simulink model "ES105A_StHlthSigNormn"  (R2013b)
settings: Solver=FixedStepDiscrete  SolverMode=SingleTasking  StartTime=0.0  StopTime=1  FixedStep=0.002  RelTol=1e-3
undefined symbols (not defined in the file): ARCHGLBPRM_FLOATZEROTHD_ULS_F32, CurrMeasCorrlnMaxErrCurr, CURRMOTSUMDIVBYZEROPROTNVAL_AMPR_F32, DIGTQDIVBYZEROPROTNVAL_HWNWTMTR_F32, DutyCycThermProtnDutyCycFildThd, EcuTMeasRngDiagcMax, EcuTMeasRngDiagcMin, EotLrngAuthyStrtLrn, FRICESTIMNDIVBYZEROPROTNVAL_HWNWTMTR_F32, HLTH0PERC_CNT_U08, HLTH100PERC_CNT_F32, HLTH100PERC_CNT_U08, HLTH50PERC_CNT_U08, HwTqCorrlnChATraSumSetFltThd, HwTqCorrlnChBTraSumSetFltThd, HWTQIDPTSIG_CNT_U08, MOTAG2MEAS_VALMAXERR_VOLTSQD_F32, MOTAG2MEAS_VALMINERR_VOLTSQD_F32, MOTAGCORRLN_MOTAGCORRLNERRTHD_MOTREVELEC_U0P16, MotDrvDiagcErrThd, MOTPOS2DIVBYZEROPROTNVAL2_VOLTSQD_F32, MOTPOS2DIVBYZEROPROTNVAL_VOLTSQD_F32, MOTPOSNERRDIVBYZEROPROTNVAL_MOTREV_U16, MOTPOSNERRZEROTHD_MOTREV_U0P16, NtcNr1, NtcSts1, PHAVLTGDIVBYZEROPROTNVAL_NANOSEC_F32, SigQlfr1, STHLTHSCAGFAC_CNT_F32, StHlthSigNormnAbsltMotPosDifStHlthDiagThd, StHlthSigNormnCurrMotSumStHlthDiagThd, StHlthSigNormnDigTqStHlthDiagThd, StHlthSigNormnDutyCycFltLimThd, StHlthSigNormnHiCtrlrT, StHlthSigNormnIdptSigStHlthSca, StHlthSigNormnLoCtrlrT, StHlthSigNormnMaxFricThd, StHlthSigNormnMinRackTrvlLim, StHlthSigNormnMotPosStHlthDiagThd, StHlthSigNormnMotVelCal, StHlthSigNormnPhaInfoStHlthDiagThd, StHlthSigNormnStHlthCorrlnErr, StHlthSigNormnStHlthCurrMotSum, StHlthSigNormnStHlthPhaInfo, StHlthSigNormnValMaxStHlthErr, StHlthSigNormnValMinStHlthErr, StHlthSigNormnWhlImbRejctnThd, SysGlbPrmMotPoleCnt, TSTHLTH0PERC_CNT_U08, u2, u3, u4, VLTGSTHLTH0PERC_CNT_U08
libraries: NxtrLim x39, simulink x33, NxtrAbslt x4
(part 7 of 10)

== system ES105A_StHlthSigNormn/StHlthSigNormn/UpdRawSig/Phase Voltage Verification/PhaBStHlth Calc/If Action Subsystem5 ==
  Action Port : ActionPort  ActionType=else
  Constant : Constant  Value=HLTH100PERC_CNT_U08
  CopyRight2 : Subsystem  Description=|  mask(Copyright Information){none=on}
      | Copyright info block.                                               
      |                                                                     
      | Place copyright information at the top of every subsystem in design.
      mask prompts: none "No parameters"
      mask help: Place copyright information at the top of every subsystem in design.
      mask Display:
      | NxtrConf = 'Nexteer Confidential';
      | 
      | sys = bdroot; %handle for the current model ("system")
      | first = get_param(sys,'Created');
      | first = first(end-3:end);  %year is last four digits
      | 
      | last = get_param(sys,'LastModifiedDate');
      | if isempty(last)
      |     last = datestr(now,'yyyy');
      | else
      |     last = last(end-3:end);
      | end
      | 
      | if strcmp(first,last)
      |     fprintf('%s -- Copyright %s Nexteer',NxtrConf,first)
      | else
      |     fprintf('%s -- %s%s- %s Nexteer',NxtrConf,char(169),first,last)
      | end
  PhaseAStHlth : Outport
  wires:
  Constant/1 -> PhaseAStHlth/1

== system ES105A_StHlthSigNormn/StHlthSigNormn/UpdRawSig/Phase Voltage Verification/PhaCStHlth Calc/CopyRight2 ==

== system ES105A_StHlthSigNormn/StHlthSigNormn/UpdRawSig/Phase Voltage Verification/PhaCStHlth Calc/If Action Subsystem8 ==
  MotDrvErrC : Inport
  Action Port : ActionPort  ActionType=then
  Constant : Constant  Value=MotDrvDiagcErrThd
  CopyRight2 : Subsystem  Description=|  mask(Copyright Information){none=on}
      | Copyright info block.                                               
      |                                                                     
      | Place copyright information at the top of every subsystem in design.
      mask prompts: none "No parameters"
      mask help: Place copyright information at the top of every subsystem in design.
      mask Display:
      | NxtrConf = 'Nexteer Confidential';
      | 
      | sys = bdroot; %handle for the current model ("system")
      | first = get_param(sys,'Created');
      | first = first(end-3:end);  %year is last four digits
      | 
      | last = get_param(sys,'LastModifiedDate');
      | if isempty(last)
      |     last = datestr(now,'yyyy');
      | else
      |     last = last(end-3:end);
      | end
      | 
      | if strcmp(first,last)
      |     fprintf('%s -- Copyright %s Nexteer',NxtrConf,first)
      | else
      |     fprintf('%s -- %s%s- %s Nexteer',NxtrConf,char(169),first,last)
      | end
  If : If  IfExpression=u1
  If Action Subsystem : Subsystem  TreatAsAtomicUnit=on
  If Action Subsystem1 : Subsystem  TreatAsAtomicUnit=on
  Merge : Merge
  Relational Operator : RelationalOperator  OutDataTypeStr=boolean
  PhaseCStHlth : Outport
  wires:
  MotDrvErrC/1 -> [MotDrvErrC], Relational Operator/1
  Constant/1 -> Relational Operator/2
  Relational Operator/1 -> If/1
  If/1 -> If Action Subsystem/Action
  If/2 -> If Action Subsystem1/Action
  [MotDrvErrC] -> If Action Subsystem1/1(MotDrvErrC)
  If Action Subsystem/1(PhaseCStHlth) -> Merge/1
  If Action Subsystem1/1(PhaseCStHlth) -> Merge/2
  Merge/1 -> PhaseCStHlth/1

== system ES105A_StHlthSigNormn/StHlthSigNormn/UpdRawSig/Phase Voltage Verification/PhaCStHlth Calc/If Action Subsystem9 ==
  Action Port : ActionPort  ActionType=else
  Constant : Constant  Value=HLTH100PERC_CNT_U08
  CopyRight2 : Subsystem  Description=|  mask(Copyright Information){none=on}
      | Copyright info block.                                               
      |                                                                     
      | Place copyright information at the top of every subsystem in design.
      mask prompts: none "No parameters"
      mask help: Place copyright information at the top of every subsystem in design.
      mask Display:
      | NxtrConf = 'Nexteer Confidential';
      | 
      | sys = bdroot; %handle for the current model ("system")
      | first = get_param(sys,'Created');
      | first = first(end-3:end);  %year is last four digits
      | 
      | last = get_param(sys,'LastModifiedDate');
      | if isempty(last)
      |     last = datestr(now,'yyyy');
      | else
      |     last = last(end-3:end);
      | end
      | 
      | if strcmp(first,last)
      |     fprintf('%s -- Copyright %s Nexteer',NxtrConf,first)
      | else
      |     fprintf('%s -- %s%s- %s Nexteer',NxtrConf,char(169),first,last)
      | end
  PhaseCStHlth : Outport
  wires:
  Constant/1 -> PhaseCStHlth/1

== system ES105A_StHlthSigNormn/StHlthSigNormn/UpdRawSig/Phase Voltage Verification/PhaDStHlth Calc/CopyRight2 ==

== system ES105A_StHlthSigNormn/StHlthSigNormn/UpdRawSig/Phase Voltage Verification/PhaDStHlth Calc/If Action Subsystem12 ==
  MotDrvErrD : Inport
  Action Port : ActionPort  ActionType=then
  Constant : Constant  Value=MotDrvDiagcErrThd
  CopyRight2 : Subsystem  Description=|  mask(Copyright Information){none=on}
      | Copyright info block.                                               
      |                                                                     
      | Place copyright information at the top of every subsystem in design.
      mask prompts: none "No parameters"
      mask help: Place copyright information at the top of every subsystem in design.
      mask Display:
      | NxtrConf = 'Nexteer Confidential';
      | 
      | sys = bdroot; %handle for the current model ("system")
      | first = get_param(sys,'Created');
      | first = first(end-3:end);  %year is last four digits
      | 
      | last = get_param(sys,'LastModifiedDate');
      | if isempty(last)
      |     last = datestr(now,'yyyy');
      | else
      |     last = last(end-3:end);
      | end
      | 
      | if strcmp(first,last)
      |     fprintf('%s -- Copyright %s Nexteer',NxtrConf,first)
      | else
      |     fprintf('%s -- %s%s- %s Nexteer',NxtrConf,char(169),first,last)
      | end
  If : If  IfExpression=u1
  If Action Subsystem : Subsystem  TreatAsAtomicUnit=on
  If Action Subsystem1 : Subsystem  TreatAsAtomicUnit=on
  Merge : Merge
  Relational Operator : RelationalOperator  OutDataTypeStr=boolean
  PhaseDStHlth : Outport
  wires:
  MotDrvErrD/1 -> [MotDrvErrD], Relational Operator/1
  Constant/1 -> Relational Operator/2
  Relational Operator/1 -> If/1
  If/1 -> If Action Subsystem/Action
  If/2 -> If Action Subsystem1/Action
  [MotDrvErrD] -> If Action Subsystem1/1(MotDrvErrD)
  If Action Subsystem/1(PhaseDStHlth) -> Merge/1
  If Action Subsystem1/1(PhaseDStHlth) -> Merge/2
  Merge/1 -> PhaseDStHlth/1

== system ES105A_StHlthSigNormn/StHlthSigNormn/UpdRawSig/Phase Voltage Verification/PhaDStHlth Calc/If Action Subsystem13 ==
  Action Port : ActionPort  ActionType=else
  Constant : Constant  Value=HLTH100PERC_CNT_U08
  CopyRight2 : Subsystem  Description=|  mask(Copyright Information){none=on}
      | Copyright info block.                                               
      |                                                                     
      | Place copyright information at the top of every subsystem in design.
      mask prompts: none "No parameters"
      mask help: Place copyright information at the top of every subsystem in design.
      mask Display:
      | NxtrConf = 'Nexteer Confidential';
      | 
      | sys = bdroot; %handle for the current model ("system")
      | first = get_param(sys,'Created');
      | first = first(end-3:end);  %year is last four digits
      | 
      | last = get_param(sys,'LastModifiedDate');
      | if isempty(last)
      |     last = datestr(now,'yyyy');
      | else
      |     last = last(end-3:end);
      | end
      | 
      | if strcmp(first,last)
      |     fprintf('%s -- Copyright %s Nexteer',NxtrConf,first)
      | else
      |     fprintf('%s -- %s%s- %s Nexteer',NxtrConf,char(169),first,last)
      | end
  PhaseDStHlth : Outport
  wires:
  Constant/1 -> PhaseDStHlth/1

== system ES105A_StHlthSigNormn/StHlthSigNormn/UpdRawSig/Phase Voltage Verification/PhaEStHlth Calc/CopyRight2 ==

== system ES105A_StHlthSigNormn/StHlthSigNormn/UpdRawSig/Phase Voltage Verification/PhaEStHlth Calc/If Action Subsystem16 ==
  MotDrvErrE : Inport
  Action Port : ActionPort  ActionType=then
  Constant : Constant  Value=MotDrvDiagcErrThd
  CopyRight2 : Subsystem  Description=|  mask(Copyright Information){none=on}
      | Copyright info block.                                               
      |                                                                     
      | Place copyright information at the top of every subsystem in design.
      mask prompts: none "No parameters"
      mask help: Place copyright information at the top of every subsystem in design.
      mask Display:
      | NxtrConf = 'Nexteer Confidential';
      | 
      | sys = bdroot; %handle for the current model ("system")
      | first = get_param(sys,'Created');
      | first = first(end-3:end);  %year is last four digits
      | 
      | last = get_param(sys,'LastModifiedDate');
      | if isempty(last)
      |     last = datestr(now,'yyyy');
      | else
      |     last = last(end-3:end);
      | end
      | 
      | if strcmp(first,last)
      |     fprintf('%s -- Copyright %s Nexteer',NxtrConf,first)
      | else
      |     fprintf('%s -- %s%s- %s Nexteer',NxtrConf,char(169),first,last)
      | end
  If : If  IfExpression=u1
  If Action Subsystem : Subsystem  TreatAsAtomicUnit=on
  If Action Subsystem1 : Subsystem  TreatAsAtomicUnit=on
  Merge : Merge
  Relational Operator : RelationalOperator  OutDataTypeStr=boolean
  PhaseEStHlth : Outport
  wires:
  MotDrvErrE/1 -> [MotDrvErrE], Relational Operator/1
  Constant/1 -> Relational Operator/2
  Relational Operator/1 -> If/1
  If/1 -> If Action Subsystem/Action
  If/2 -> If Action Subsystem1/Action
  [MotDrvErrE] -> If Action Subsystem1/1(MotDrvErrE)
  If Action Subsystem/1(PhaseEStHlth) -> Merge/1
  If Action Subsystem1/1(PhaseEStHlth) -> Merge/2
  Merge/1 -> PhaseEStHlth/1

== system ES105A_StHlthSigNormn/StHlthSigNormn/UpdRawSig/Phase Voltage Verification/PhaEStHlth Calc/If Action Subsystem17 ==
  Action Port : ActionPort  ActionType=else
  Constant : Constant  Value=HLTH100PERC_CNT_U08
  CopyRight2 : Subsystem  Description=|  mask(Copyright Information){none=on}
      | Copyright info block.                                               
      |                                                                     
      | Place copyright information at the top of every subsystem in design.
      mask prompts: none "No parameters"
      mask help: Place copyright information at the top of every subsystem in design.
      mask Display:
      | NxtrConf = 'Nexteer Confidential';
      | 
      | sys = bdroot; %handle for the current model ("system")
      | first = get_param(sys,'Created');
      | first = first(end-3:end);  %year is last four digits
      | 
      | last = get_param(sys,'LastModifiedDate');
      | if isempty(last)
      |     last = datestr(now,'yyyy');
      | else
      |     last = last(end-3:end);
      | end
      | 
      | if strcmp(first,last)
      |     fprintf('%s -- Copyright %s Nexteer',NxtrConf,first)
      | else
      |     fprintf('%s -- %s%s- %s Nexteer',NxtrConf,char(169),first,last)
      | end
  PhaseEStHlth : Outport
  wires:
  Constant/1 -> PhaseEStHlth/1

== system ES105A_StHlthSigNormn/StHlthSigNormn/UpdRawSig/Phase Voltage Verification/PhaFStHlth Calc/CopyRight2 ==

== system ES105A_StHlthSigNormn/StHlthSigNormn/UpdRawSig/Phase Voltage Verification/PhaFStHlth Calc/If Action Subsystem20 ==
  MotDrvErrF : Inport
  Action Port : ActionPort  ActionType=then
  Constant : Constant  Value=MotDrvDiagcErrThd
  CopyRight2 : Subsystem  Description=|  mask(Copyright Information){none=on}
      | Copyright info block.                                               
      |                                                                     
      | Place copyright information at the top of every subsystem in design.
      mask prompts: none "No parameters"
      mask help: Place copyright information at the top of every subsystem in design.
      mask Display:
      | NxtrConf = 'Nexteer Confidential';
      | 
      | sys = bdroot; %handle for the current model ("system")
      | first = get_param(sys,'Created');
      | first = first(end-3:end);  %year is last four digits
      | 
      | last = get_param(sys,'LastModifiedDate');
      | if isempty(last)
      |     last = datestr(now,'yyyy');
      | else
      |     last = last(end-3:end);
      | end
      | 
      | if strcmp(first,last)
      |     fprintf('%s -- Copyright %s Nexteer',NxtrConf,first)
      | else
      |     fprintf('%s -- %s%s- %s Nexteer',NxtrConf,char(169),first,last)
      | end
  If : If  IfExpression=u1
  If Action Subsystem : Subsystem  TreatAsAtomicUnit=on
  If Action Subsystem1 : Subsystem  TreatAsAtomicUnit=on
  Merge : Merge
  Relational Operator : RelationalOperator  OutDataTypeStr=boolean
  PhaseFStHlth : Outport
  wires:
  MotDrvErrF/1 -> [MotDrvErrF], Relational Operator/1
  Constant/1 -> Relational Operator/2
  Relational Operator/1 -> If/1
  If/1 -> If Action Subsystem/Action
  If/2 -> If Action Subsystem1/Action
  [MotDrvErrF] -> If Action Subsystem1/1(MotDrvErrF)
  If Action Subsystem/1(PhaseFStHlth) -> Merge/1
  If Action Subsystem1/1(PhaseFStHlth) -> Merge/2
  Merge/1 -> PhaseFStHlth/1

== system ES105A_StHlthSigNormn/StHlthSigNormn/UpdRawSig/Phase Voltage Verification/PhaFStHlth Calc/If Action Subsystem21 ==
  Action Port : ActionPort  ActionType=else
  Constant : Constant  Value=HLTH100PERC_CNT_U08
  CopyRight2 : Subsystem  Description=|  mask(Copyright Information){none=on}
      | Copyright info block.                                               
      |                                                                     
      | Place copyright information at the top of every subsystem in design.
      mask prompts: none "No parameters"
      mask help: Place copyright information at the top of every subsystem in design.
      mask Display:
      | NxtrConf = 'Nexteer Confidential';
      | 
      | sys = bdroot; %handle for the current model ("system")
      | first = get_param(sys,'Created');
      | first = first(end-3:end);  %year is last four digits
      | 
      | last = get_param(sys,'LastModifiedDate');
      | if isempty(last)
      |     last = datestr(now,'yyyy');
      | else
      |     last = last(end-3:end);
      | end
      | 
      | if strcmp(first,last)
      |     fprintf('%s -- Copyright %s Nexteer',NxtrConf,first)
      | else
      |     fprintf('%s -- %s%s- %s Nexteer',NxtrConf,char(169),first,last)
      | end
  PhaseFStHlth : Outport
  wires:
  Constant/1 -> PhaseFStHlth/1

== system ES105A_StHlthSigNormn/StHlthSigNormn/UpdRawSig/Phase Voltage Verification/PhaStHlth/SetNtcSts ==
  note: Note:
      |
      | - "ISO Fault Debounce Design" Simulink block intent to use here for Simulation purpose only. Do not Code this block
  NtcNr : Inport
  NtcStInfo : Inport  Port=2
  NtcSts : Inport  Port=3
  DebStep : Inport  Port=4
  CopyRight2 : Subsystem  Description=|  mask(Copyright Information){none=on}
      | Copyright info block.                                               
      |                                                                     
      | Place copyright information at the top of every subsystem in design.
      mask prompts: none "No parameters"
      mask help: Place copyright information at the top of every subsystem in design.
      mask Display:
      | NxtrConf = 'Nexteer Confidential';
      | 
      | sys = bdroot; %handle for the current model ("system")
      | first = get_param(sys,'Created');
      | first = first(end-3:end);  %year is last four digits
      | 
      | last = get_param(sys,'LastModifiedDate');
      | if isempty(last)
      |     last = datestr(now,'yyyy');
      | else
      |     last = last(end-3:end);
      | end
      | 
      | if strcmp(first,last)
      |     fprintf('%s -- Copyright %s Nexteer',NxtrConf,first)
      | else
      |     fprintf('%s -- %s%s- %s Nexteer',NxtrConf,char(169),first,last)
      | end
  Data Store Write : DataStoreWrite  DataStoreName=NtcQlfr0X1D4
  Ground : Ground
  ISO Fault Debounce Design : Stateflow chart  TreatAsAtomicUnit=on
      settings: AttributesFormatString=|
      | Simulation Purpose Only.
      | Do Not Code this block
      | Diagnostic Manager Owns this requirement
  Terminator : Terminator
  Terminator1 : Terminator
  wires:
  NtcStInfo/1 -> Terminator1/1
  NtcNr/1 -> Terminator/1
  NtcSts/1 -> ISO Fault Debounce Design/1(NtcSts)
  DebStep/1 -> ISO Fault Debounce Design/2(DebStep)
  ISO Fault Debounce Design/1(Qualifier) -> Data Store Write/1
  Ground/1 -> ISO Fault Debounce Design/3(SvcClr)

== system ES105A_StHlthSigNormn/StHlthSigNormn/UpdRawSig/Wheel Imbalance Rejection/If Action Subsystem/CopyRight2 ==

== system ES105A_StHlthSigNormn/StHlthSigNormn/UpdRawSig/Wheel Imbalance Rejection/If Action Subsystem2/CopyRight2 ==

== system ES105A_StHlthSigNormn/StHlthSigNormn/UpdRawSig/ EOT Impact Counter/If Action Subsystem/If Action Subsystem/CopyRight2 ==

== system ES105A_StHlthSigNormn/StHlthSigNormn/UpdRawSig/ EOT Impact Counter/If Action Subsystem/If Action Subsystem/If Action Subsystem ==
  "MotVelCrf " : Inport
  Action Port : ActionPort  ActionType=then
  Constant : Constant  Value=StHlthSigNormnMotVelCal
  CopyRight2 : Subsystem  Description=|  mask(Copyright Information){none=on}
      | Copyright info block.                                               
      |                                                                     
      | Place copyright information at the top of every subsystem in design.
      mask prompts: none "No parameters"
      mask help: Place copyright information at the top of every subsystem in design.
      mask Display:
      | NxtrConf = 'Nexteer Confidential';
      | 
      | sys = bdroot; %handle for the current model ("system")
      | first = get_param(sys,'Created');
      | first = first(end-3:end);  %year is last four digits
      | 
      | last = get_param(sys,'LastModifiedDate');
      | if isempty(last)
      |     last = datestr(now,'yyyy');
      | else
      |     last = last(end-3:end);
      | end
      | 
      | if strcmp(first,last)
      |     fprintf('%s -- Copyright %s Nexteer',NxtrConf,first)
      | else
      |     fprintf('%s -- %s%s- %s Nexteer',NxtrConf,char(169),first,last)
      | end
  Do nothing : Subsystem  TreatAsAtomicUnit=on
  If : If  IfExpression=u1
  If Action Subsystem : Subsystem  TreatAsAtomicUnit=on
  Relational Operator1 : RelationalOperator  Operator=>  OutDataTypeStr=boolean
  wires:
  "MotVelCrf "/1 -> Relational Operator1/1
  Constant/1 -> Relational Operator1/2
  Relational Operator1/1 -> If/1
  If/1 -> If Action Subsystem/Action
  If/2 -> Do nothing/Action

== system ES105A_StHlthSigNormn/StHlthSigNormn/UpdRawSig/ EOT Impact Counter/If Action Subsystem/If Action Subsystem/If Action Subsystem1 ==
  Action Port : ActionPort  ActionType=else
  Constant : Constant  Value=0  OutDataTypeStr=boolean
      settings: AttributesFormatString=%<OutDataTypeStr>
  CopyRight2 : Subsystem  Description=|  mask(Copyright Information){none=on}
      | Copyright info block.                                               
      |                                                                     
      | Place copyright information at the top of every subsystem in design.
      mask prompts: none "No parameters"
      mask help: Place copyright information at the top of every subsystem in design.
      mask Display:
      | NxtrConf = 'Nexteer Confidential';
      | 
      | sys = bdroot; %handle for the current model ("system")
      | first = get_param(sys,'Created');
      | first = first(end-3:end);  %year is last four digits
      | 
      | last = get_param(sys,'LastModifiedDate');
      | if isempty(last)
      |     last = datestr(now,'yyyy');
      | else
      |     last = last(end-3:end);
      | end
      | 
      | if strcmp(first,last)
      |     fprintf('%s -- Copyright %s Nexteer',NxtrConf,first)
      | else
      |     fprintf('%s -- %s%s- %s Nexteer',NxtrConf,char(169),first,last)
      | end
  Data Store Write : DataStoreWrite  DataStoreName=EntrEot
  wires:
  Constant/1 -> Data Store Write/1

== system ES105A_StHlthSigNormn/StHlthSigNormn/UpdRawSig/ EOT Impact Counter/If Action Subsystem/If Action Subsystem1/CopyRight2 ==

== system ES105A_StHlthSigNormn/StHlthSigNormn/UpdRawSig/ EOT Impact Counter/If Action Subsystem/If Action Subsystem1/If Action Subsystem ==
  "MotVelCrf " : Inport
  Action Port : ActionPort  ActionType=then
  Constant : Constant  Value=StHlthSigNormnMotVelCal
  CopyRight2 : Subsystem  Description=|  mask(Copyright Information){none=on}
      | Copyright info block.                                               
      |                                                                     
      | Place copyright information at the top of every subsystem in design.
      mask prompts: none "No parameters"
      mask help: Place copyright information at the top of every subsystem in design.
      mask Display:
      | NxtrConf = 'Nexteer Confidential';
      | 
      | sys = bdroot; %handle for the current model ("system")
      | first = get_param(sys,'Created');
      | first = first(end-3:end);  %year is last four digits
      | 
      | last = get_param(sys,'LastModifiedDate');
      | if isempty(last)
      |     last = datestr(now,'yyyy');
      | else
      |     last = last(end-3:end);
      | end
      | 
      | if strcmp(first,last)
      |     fprintf('%s -- Copyright %s Nexteer',NxtrConf,first)
      | else
      |     fprintf('%s -- %s%s- %s Nexteer',NxtrConf,char(169),first,last)
      | end
  Do nothing : Subsystem  TreatAsAtomicUnit=on
  If : If  IfExpression=u1
  If Action Subsystem : Subsystem  TreatAsAtomicUnit=on
  Relational Operator1 : RelationalOperator  Operator=<  OutDataTypeStr=boolean
  Unary Minus : UnaryMinus
  wires:
  "MotVelCrf "/1 -> Relational Operator1/1
  Constant/1 -> Unary Minus/1
  Relational Operator1/1 -> If/1
  If/1 -> If Action Subsystem/Action
  Unary Minus/1 -> Relational Operator1/2
  If/2 -> Do nothing/Action

== system ES105A_StHlthSigNormn/StHlthSigNormn/UpdRawSig/ EOT Impact Counter/If Action Subsystem/If Action Subsystem1/If Action Subsystem1 ==
  Action Port : ActionPort  ActionType=else
  Constant : Constant  Value=0  OutDataTypeStr=boolean
      settings: AttributesFormatString=%<OutDataTypeStr>
  CopyRight2 : Subsystem  Description=|  mask(Copyright Information){none=on}
      | Copyright info block.                                               
      |                                                                     
      | Place copyright information at the top of every subsystem in design.
      mask prompts: none "No parameters"
      mask help: Place copyright information at the top of every subsystem in design.
      mask Display:
      | NxtrConf = 'Nexteer Confidential';
      | 
      | sys = bdroot; %handle for the current model ("system")
      | first = get_param(sys,'Created');
      | first = first(end-3:end);  %year is last four digits
      | 
      | last = get_param(sys,'LastModifiedDate');
      | if isempty(last)
      |     last = datestr(now,'yyyy');
      | else
      |     last = last(end-3:end);
      | end
      | 
      | if strcmp(first,last)
      |     fprintf('%s -- Copyright %s Nexteer',NxtrConf,first)
      | else
      |     fprintf('%s -- %s%s- %s Nexteer',NxtrConf,char(169),first,last)
      | end
  Data Store Write : DataStoreWrite  DataStoreName=EntrEot
  wires:
  Constant/1 -> Data Store Write/1

== system ES105A_StHlthSigNormn/StHlthSigNormn/UpdRawSig/Current Error/CurrMotSumABCStHlth Calc/If Action Subsystem/CopyRight2 ==

== system ES105A_StHlthSigNormn/StHlthSigNormn/UpdRawSig/Current Error/CurrMotSumABCStHlth Calc/If Action Subsystem/If Action Subsystem ==
  Action Port : ActionPort  ActionType=then
  Constant : Constant  Value=HLTH0PERC_CNT_U08  OutDataTypeStr=uint8
  CopyRight2 : Subsystem  Description=|  mask(Copyright Information){none=on}
      | Copyright info block.                                               
      |                                                                     
      | Place copyright information at the top of every subsystem in design.
      mask prompts: none "No parameters"
      mask help: Place copyright information at the top of every subsystem in design.
      mask Display:
      | NxtrConf = 'Nexteer Confidential';
      | 
      | sys = bdroot; %handle for the current model ("system")
      | first = get_param(sys,'Created');
      | first = first(end-3:end);  %year is last four digits
      | 
      | last = get_param(sys,'LastModifiedDate');
      | if isempty(last)
      |     last = datestr(now,'yyyy');
      | else
      |     last = last(end-3:end);
      | end
      | 
      | if strcmp(first,last)
      |     fprintf('%s -- Copyright %s Nexteer',NxtrConf,first)
      | else
      |     fprintf('%s -- %s%s- %s Nexteer',NxtrConf,char(169),first,last)
      | end
  CurrMotSumABCStHlth : Outport
  wires:
  Constant/1 -> CurrMotSumABCStHlth/1

== system ES105A_StHlthSigNormn/StHlthSigNormn/UpdRawSig/Current Error/CurrMotSumABCStHlth Calc/If Action Subsystem/If Action Subsystem1 ==
  CurrMotSumABC : Inport
  Action Port : ActionPort  ActionType=else
  Constant : Constant  Value=CurrMeasCorrlnMaxErrCurr
  Constant3 : Constant  Value=HLTH100PERC_CNT_U08
  CopyRight2 : Subsystem  Description=|  mask(Copyright Information){none=on}
      | Copyright info block.                                               
      |                                                                     
      | Place copyright information at the top of every subsystem in design.
      mask prompts: none "No parameters"
      mask help: Place copyright information at the top of every subsystem in design.
      mask Display:
      | NxtrConf = 'Nexteer Confidential';
      | 
      | sys = bdroot; %handle for the current model ("system")
      | first = get_param(sys,'Created');
      | first = first(end-3:end);  %year is last four digits
      | 
      | last = get_param(sys,'LastModifiedDate');
      | if isempty(last)
      |     last = datestr(now,'yyyy');
      | else
      |     last = last(end-3:end);
      | end
      | 
      | if strcmp(first,last)
      |     fprintf('%s -- Copyright %s Nexteer',NxtrConf,first)
      | else
      |     fprintf('%s -- %s%s- %s Nexteer',NxtrConf,char(169),first,last)
      | end
  Data Type Conversion : DataTypeConversion  OutDataTypeStr=uint8
  Divide : Product  Inputs=*/
  Divide by Zero Protection for Cal : Subsystem
  LimStat_f32 : NxtrLim/LimStat_f32  LoLim=STHLTHFLOATZEROVAL_ULS_F32  HiLim=STHLTHFLOATTWOFIFTYFIVEVAL_ULS_F32
      settings: AttributesFormatString=|
      | Low Limit: %<LoLim>
      | High Limit:%<HiLim>
  Product : Product
  Subtract : Sum  Inputs=+-
  CurrMotSumABCStHlth : Outport
  wires:
  Constant/1 -> Subtract/1
  CurrMotSumABC/1 -> Subtract/2
  Subtract/1 -> Divide/1
  Constant3/1 -> Product/2
  Divide/1 -> Product/1
  Divide by Zero Protection for Cal/1(CurrMotSumDelta) -> Divide/2
  LimStat_f32/1 -> Data Type Conversion/1
  Product/1 -> LimStat_f32/1
  Data Type Conversion/1 -> CurrMotSumABCStHlth/1

== system ES105A_StHlthSigNormn/StHlthSigNormn/UpdRawSig/Current Error/CurrMotSumABCStHlth Calc/If Action Subsystem1/CopyRight2 ==

== system ES105A_StHlthSigNormn/StHlthSigNormn/UpdRawSig/Current Error/CurrMotSumDEFStHlth Calc/If Action Subsystem4/CopyRight2 ==

== system ES105A_StHlthSigNormn/StHlthSigNormn/UpdRawSig/Current Error/CurrMotSumDEFStHlth Calc/If Action Subsystem4/If Action Subsystem ==
  Action Port : ActionPort  ActionType=then
  Constant : Constant  Value=HLTH0PERC_CNT_U08  OutDataTypeStr=uint8
  CopyRight2 : Subsystem  Description=|  mask(Copyright Information){none=on}
      | Copyright info block.                                               
      |                                                                     
      | Place copyright information at the top of every subsystem in design.
      mask prompts: none "No parameters"
      mask help: Place copyright information at the top of every subsystem in design.
      mask Display:
      | NxtrConf = 'Nexteer Confidential';
      | 
      | sys = bdroot; %handle for the current model ("system")
      | first = get_param(sys,'Created');
      | first = first(end-3:end);  %year is last four digits
      | 
      | last = get_param(sys,'LastModifiedDate');
      | if isempty(last)
      |     last = datestr(now,'yyyy');
      | else
      |     last = last(end-3:end);
      | end
      | 
      | if strcmp(first,last)
      |     fprintf('%s -- Copyright %s Nexteer',NxtrConf,first)
      | else
      |     fprintf('%s -- %s%s- %s Nexteer',NxtrConf,char(169),first,last)
      | end
  CurrMotSumDEFStHlth : Outport
  wires:
  Constant/1 -> CurrMotSumDEFStHlth/1

== system ES105A_StHlthSigNormn/StHlthSigNormn/UpdRawSig/Current Error/CurrMotSumDEFStHlth Calc/If Action Subsystem4/If Action Subsystem1 ==
  CurrMotSumDEF : Inport
  Action Port : ActionPort  ActionType=else
  Constant : Constant  Value=CurrMeasCorrlnMaxErrCurr
  Constant3 : Constant  Value=HLTH100PERC_CNT_U08
  CopyRight2 : Subsystem  Description=|  mask(Copyright Information){none=on}
      | Copyright info block.                                               
      |                                                                     
      | Place copyright information at the top of every subsystem in design.
      mask prompts: none "No parameters"
      mask help: Place copyright information at the top of every subsystem in design.
      mask Display:
      | NxtrConf = 'Nexteer Confidential';
      | 
      | sys = bdroot; %handle for the current model ("system")
      | first = get_param(sys,'Created');
      | first = first(end-3:end);  %year is last four digits
      | 
      | last = get_param(sys,'LastModifiedDate');
      | if isempty(last)
      |     last = datestr(now,'yyyy');
      | else
      |     last = last(end-3:end);
      | end
      | 
      | if strcmp(first,last)
      |     fprintf('%s -- Copyright %s Nexteer',NxtrConf,first)
      | else
      |     fprintf('%s -- %s%s- %s Nexteer',NxtrConf,char(169),first,last)
      | end
  Data Type Conversion : DataTypeConversion  OutDataTypeStr=uint8
  Divide : Product  Inputs=*/
  Divide by Zero Protection for Cal : Subsystem
  LimStat_f32 : NxtrLim/LimStat_f32  LoLim=STHLTHFLOATZEROVAL_ULS_F32  HiLim=STHLTHFLOATTWOFIFTYFIVEVAL_ULS_F32
      settings: AttributesFormatString=|
      | Low Limit: %<LoLim>
      | High Limit:%<HiLim>
  Product : Product
  Subtract : Sum  Inputs=+-
  CurrMotSumDEFStHlth : Outport
  wires:
  Constant/1 -> Subtract/1
  CurrMotSumDEF/1 -> Subtract/2
  Subtract/1 -> Divide/1
  Divide by Zero Protection for Cal/1(CurrMotSumDelta) -> Divide/2
  Constant3/1 -> Product/2
  Divide/1 -> Product/1
  LimStat_f32/1 -> Data Type Conversion/1
  Product/1 -> LimStat_f32/1
  Data Type Conversion/1 -> CurrMotSumDEFStHlth/1

== system ES105A_StHlthSigNormn/StHlthSigNormn/UpdRawSig/Current Error/CurrMotSumDEFStHlth Calc/If Action Subsystem5/CopyRight2 ==

== system ES105A_StHlthSigNormn/StHlthSigNormn/UpdRawSig/Current Error/CurrMotSumPhaStHlth/SetNtcSts/CopyRight2 ==

== system ES105A_StHlthSigNormn/StHlthSigNormn/UpdRawSig/Current Error/NTC Sts Calculation/NtcFaild/CopyRight2 ==

== system ES105A_StHlthSigNormn/StHlthSigNormn/UpdRawSig/Current Error/NTC Sts Calculation/NtcPassd/CopyRight2 ==

== system ES105A_StHlthSigNormn/StHlthSigNormn/UpdRawSig/Digital Torque Sensor /DigTqIdptSigStHlth Calc/If Action Subsystem4/CopyRight2 ==

== system ES105A_StHlthSigNormn/StHlthSigNormn/UpdRawSig/Digital Torque Sensor /DigTqIdptSigStHlth Calc/If Action Subsystem5/CopyRight2 ==

== system ES105A_StHlthSigNormn/StHlthSigNormn/UpdRawSig/Digital Torque Sensor /DigTqSnsrAStHlth Calc/If Action Subsystem/CopyRight2 ==

== system ES105A_StHlthSigNormn/StHlthSigNormn/UpdRawSig/Digital Torque Sensor /DigTqSnsrAStHlth Calc/If Action Subsystem1/CopyRight2 ==

== system ES105A_StHlthSigNormn/StHlthSigNormn/UpdRawSig/Digital Torque Sensor /DigTqSnsrAStHlth Calc/If Action Subsystem1/Devide by Zero Protection for Cal ==
  note: Min-Max of HwTqCorrlnChATraSumSetFltThd is 0 to 20
      | There is a possibility of Divide by Zero Error.
  Constant : Constant  Value=ARCHGLBPRM_FLOATZEROTHD_ULS_F32
  Constant2 : Constant  Value=HwTqCorrlnChATraSumSetFltThd
  CopyRight2 : Subsystem  Description=|  mask(Copyright Information){none=on}
      | Copyright info block.                                               
      |                                                                     
      | Place copyright information at the top of every subsystem in design.
      mask prompts: none "No parameters"
      mask help: Place copyright information at the top of every subsystem in design.
      mask Display:
      | NxtrConf = 'Nexteer Confidential';
      | 
      | sys = bdroot; %handle for the current model ("system")
      | first = get_param(sys,'Created');
      | first = first(end-3:end);  %year is last four digits
      | 
      | last = get_param(sys,'LastModifiedDate');
      | if isempty(last)
      |     last = datestr(now,'yyyy');
      | else
      |     last = last(end-3:end);
      | end
      | 
      | if strcmp(first,last)
      |     fprintf('%s -- Copyright %s Nexteer',NxtrConf,first)
      | else
      |     fprintf('%s -- %s%s- %s Nexteer',NxtrConf,char(169),first,last)
      | end
  If : If  IfExpression=u1
  If Zero : Subsystem  TreatAsAtomicUnit=on
  Merge : Merge
  Non Zero : Subsystem  TreatAsAtomicUnit=on
  Relational Operator : RelationalOperator  Operator=<=  OutDataTypeStr=boolean
  HwTqCorrlnChATraSumSetFltThd : Outport
  wires:
  If/1 -> If Zero/Action
  If/2 -> Non Zero/Action
  Constant2/1 -> Non Zero/1(In1), Relational Operator/1
  If Zero/1(Out1) -> Merge/1
  Non Zero/1(Out1) -> Merge/2
  Merge/1 -> HwTqCorrlnChATraSumSetFltThd/1
  Relational Operator/1 -> If/1
  Constant/1 -> Relational Operator/2

== system ES105A_StHlthSigNormn/StHlthSigNormn/UpdRawSig/Digital Torque Sensor /DigTqSnsrBStHlth Calc/If Action Subsystem2/CopyRight2 ==

== system ES105A_StHlthSigNormn/StHlthSigNormn/UpdRawSig/Digital Torque Sensor /DigTqSnsrBStHlth Calc/If Action Subsystem3/CopyRight2 ==

== system ES105A_StHlthSigNormn/StHlthSigNormn/UpdRawSig/Digital Torque Sensor /DigTqSnsrBStHlth Calc/If Action Subsystem3/Devide by Zero Protection for Cal ==
  note: Min-Max of HwTqCorrlnChBTraSumSetFltThd is 0 to 20
      | There is a possibility of Divide by Zero Error.
  Constant : Constant  Value=ARCHGLBPRM_FLOATZEROTHD_ULS_F32
  Constant1 : Constant  Value=HwTqCorrlnChBTraSumSetFltThd
  CopyRight2 : Subsystem  Description=|  mask(Copyright Information){none=on}
      | Copyright info block.                                               
      |                                                                     
      | Place copyright information at the top of every subsystem in design.
      mask prompts: none "No parameters"
      mask help: Place copyright information at the top of every subsystem in design.
      mask Display:
      | NxtrConf = 'Nexteer Confidential';
      | 
      | sys = bdroot; %handle for the current model ("system")
      | first = get_param(sys,'Created');
      | first = first(end-3:end);  %year is last four digits
      | 
      | last = get_param(sys,'LastModifiedDate');
      | if isempty(last)
      |     last = datestr(now,'yyyy');
      | else
      |     last = last(end-3:end);
      | end
      | 
      | if strcmp(first,last)
      |     fprintf('%s -- Copyright %s Nexteer',NxtrConf,first)
      | else
      |     fprintf('%s -- %s%s- %s Nexteer',NxtrConf,char(169),first,last)
      | end
  If : If  IfExpression=u1
  If Zero : Subsystem  TreatAsAtomicUnit=on
  Merge : Merge
  Non Zero : Subsystem  TreatAsAtomicUnit=on
  Relational Operator : RelationalOperator  Operator=<=  OutDataTypeStr=boolean
  HwTqCorrlnChBTraSumSetFltThd : Outport
  wires:
  If/1 -> If Zero/Action
  If/2 -> Non Zero/Action
  Constant1/1 -> Non Zero/1(In1), Relational Operator/1
  If Zero/1(Out1) -> Merge/1
  Non Zero/1(Out1) -> Merge/2
  Merge/1 -> HwTqCorrlnChBTraSumSetFltThd/1
  Relational Operator/1 -> If/1
  Constant/1 -> Relational Operator/2

== system ES105A_StHlthSigNormn/StHlthSigNormn/UpdRawSig/Digital Torque Sensor /DigTqSnsrPhaStHlth/SetNtcSts/CopyRight2 ==

== system ES105A_StHlthSigNormn/StHlthSigNormn/UpdRawSig/Digital Torque Sensor /NTC Sts Calculation/NtcFaild/CopyRight2 ==

== system ES105A_StHlthSigNormn/StHlthSigNormn/UpdRawSig/Digital Torque Sensor /NTC Sts Calculation/NtcPassd/CopyRight2 ==

== system ES105A_StHlthSigNormn/StHlthSigNormn/UpdRawSig/Friction Estimation/If Action Subsystem4/Divide by Zero Protection for Cal/CopyRight2 ==

== system ES105A_StHlthSigNormn/StHlthSigNormn/UpdRawSig/Friction Estimation/If Action Subsystem4/Divide by Zero Protection for Cal/If Zero ==
  Action Port : ActionPort  ActionType=then
  Constant : Constant  Value=FRICESTIMNDIVBYZEROPROTNVAL_HWNWTMTR_F32
  CopyRight2 : Subsystem  Description=|  mask(Copyright Information){none=on}
      | Copyright info block.                                               
      |                                                                     
      | Place copyright information at the top of every subsystem in design.
      mask prompts: none "No parameters"
      mask help: Place copyright information at the top of every subsystem in design.
      mask Display:
      | NxtrConf = 'Nexteer Confidential';
      | 
      | sys = bdroot; %handle for the current model ("system")
      | first = get_param(sys,'Created');
      | first = first(end-3:end);  %year is last four digits
      | 
      | last = get_param(sys,'LastModifiedDate');
      | if isempty(last)
      |     last = datestr(now,'yyyy');
      | else
      |     last = last(end-3:end);
      | end
      | 
      | if strcmp(first,last)
      |     fprintf('%s -- Copyright %s Nexteer',NxtrConf,first)
      | else
      |     fprintf('%s -- %s%s- %s Nexteer',NxtrConf,char(169),first,last)
      | end
  Out1 : Outport
  wires:
  Constant/1 -> Out1/1

== system ES105A_StHlthSigNormn/StHlthSigNormn/UpdRawSig/Friction Estimation/If Action Subsystem4/Divide by Zero Protection for Cal/Non Zero ==
  In1 : Inport
  Action Port : ActionPort  ActionType=else
  CopyRight2 : Subsystem  Description=|  mask(Copyright Information){none=on}
      | Copyright info block.                                               
      |                                                                     
      | Place copyright information at the top of every subsystem in design.
      mask prompts: none "No parameters"
      mask help: Place copyright information at the top of every subsystem in design.
      mask Display:
      | NxtrConf = 'Nexteer Confidential';
      | 
      | sys = bdroot; %handle for the current model ("system")
      | first = get_param(sys,'Created');
      | first = first(end-3:end);  %year is last four digits
      | 
      | last = get_param(sys,'LastModifiedDate');
      | if isempty(last)
      |     last = datestr(now,'yyyy');
      | else
      |     last = last(end-3:end);
      | end
      | 
      | if strcmp(first,last)
      |     fprintf('%s -- Copyright %s Nexteer',NxtrConf,first)
      | else
      |     fprintf('%s -- %s%s- %s Nexteer',NxtrConf,char(169),first,last)
      | end
  Out1 : Outport
  wires:
  In1/1 -> Out1/1

== system ES105A_StHlthSigNormn/StHlthSigNormn/UpdRawSig/Motor Position 2 /If Action Subsystem/If Action Subsystem/CopyRight2 ==

== system ES105A_StHlthSigNormn/StHlthSigNormn/UpdRawSig/Motor Position 2 /If Action Subsystem/If Action Subsystem1/CopyRight2 ==

== system ES105A_StHlthSigNormn/StHlthSigNormn/UpdRawSig/Motor Position 2 /If Action Subsystem/If Action Subsystem1/Divide by Zero Protection for Cal ==
  note: Eliminate Divide by Zero Error.
  Constant : Constant  Value=ARCHGLBPRM_FLOATZEROTHD_ULS_F32
  Constant1 : Constant  Value=MOTAG2MEAS_VALMINERR_VOLTSQD_F32
  Constant2 : Constant  Value=StHlthSigNormnValMinStHlthErr
  CopyRight2 : Subsystem  Description=|  mask(Copyright Information){none=on}
      | Copyright info block.                                               
      |                                                                     
      | Place copyright information at the top of every subsystem in design.
      mask prompts: none "No parameters"
      mask help: Place copyright information at the top of every subsystem in design.
      mask Display:
      | NxtrConf = 'Nexteer Confidential';
      | 
      | sys = bdroot; %handle for the current model ("system")
      | first = get_param(sys,'Created');
      | first = first(end-3:end);  %year is last four digits
      | 
      | last = get_param(sys,'LastModifiedDate');
      | if isempty(last)
      |     last = datestr(now,'yyyy');
      | else
      |     last = last(end-3:end);
      | end
      | 
      | if strcmp(first,last)
      |     fprintf('%s -- Copyright %s Nexteer',NxtrConf,first)
      | else
      |     fprintf('%s -- %s%s- %s Nexteer',NxtrConf,char(169),first,last)
      | end
  If : If  IfExpression=u1
  If Zero : Subsystem  TreatAsAtomicUnit=on
  Merge : Merge
  Non Zero : Subsystem  TreatAsAtomicUnit=on
  Relational Operator : RelationalOperator  Operator=<=  OutDataTypeStr=boolean
  Subtract1 : Sum  Inputs=+-
  MotorPos2DeltaMin : Outport
  wires:
  If/1 -> If Zero/Action
  If/2 -> Non Zero/Action
  If Zero/1(Out1) -> Merge/1
  Non Zero/1(Out1) -> Merge/2
  Merge/1 -> MotorPos2DeltaMin/1
  Relational Operator/1 -> If/1
  Constant/1 -> Relational Operator/2
  Constant2/1 -> Subtract1/1
  Constant1/1 -> Subtract1/2
  Subtract1/1 -> Non Zero/1(In1), Relational Operator/1

== system ES105A_StHlthSigNormn/StHlthSigNormn/UpdRawSig/Motor Position 2 /If Action Subsystem/If Action Subsystem2/CopyRight2 ==

== system ES105A_StHlthSigNormn/StHlthSigNormn/UpdRawSig/Motor Position 2 /If Action Subsystem/If Action Subsystem2/Divide by Zero Protection for Cal ==
  note: Eliminate Divide by Zero Error.
  Constant : Constant  Value=ARCHGLBPRM_FLOATZEROTHD_ULS_F32
  Constant1 : Constant  Value=MOTAG2MEAS_VALMAXERR_VOLTSQD_F32
  Constant4 : Constant  Value=StHlthSigNormnValMaxStHlthErr
  CopyRight2 : Subsystem  Description=|  mask(Copyright Information){none=on}
      | Copyright info block.                                               
      |                                                                     
      | Place copyright information at the top of every subsystem in design.
      mask prompts: none "No parameters"
      mask help: Place copyright information at the top of every subsystem in design.
      mask Display:
      | NxtrConf = 'Nexteer Confidential';
      | 
      | sys = bdroot; %handle for the current model ("system")
      | first = get_param(sys,'Created');
      | first = first(end-3:end);  %year is last four digits
      | 
      | last = get_param(sys,'LastModifiedDate');
      | if isempty(last)
      |     last = datestr(now,'yyyy');
      | else
      |     last = last(end-3:end);
      | end
      | 
      | if strcmp(first,last)
      |     fprintf('%s -- Copyright %s Nexteer',NxtrConf,first)
      | else
      |     fprintf('%s -- %s%s- %s Nexteer',NxtrConf,char(169),first,last)
      | end
  If : If  IfExpression=u1
  If Zero : Subsystem  TreatAsAtomicUnit=on
  Merge : Merge
  Non Zero : Subsystem  TreatAsAtomicUnit=on
  Relational Operator : RelationalOperator  Operator=<=  OutDataTypeStr=boolean
  Subtract : Sum  Inputs=+-
  MotorPos2DeltaMax : Outport
  wires:
  If/1 -> If Zero/Action
  If/2 -> Non Zero/Action
  If Zero/1(Out1) -> Merge/1
  Non Zero/1(Out1) -> Merge/2
  Merge/1 -> MotorPos2DeltaMax/1
  Relational Operator/1 -> If/1
  Constant/1 -> Relational Operator/2
  Constant1/1 -> Subtract/1
  Constant4/1 -> Subtract/2
  Subtract/1 -> Non Zero/1(In1), Relational Operator/1

== system ES105A_StHlthSigNormn/StHlthSigNormn/UpdRawSig/Motor Position 2 /NTC Sts Calculation/NtcFaild/CopyRight2 ==

== system ES105A_StHlthSigNormn/StHlthSigNormn/UpdRawSig/Motor Position 2 /NTC Sts Calculation/NtcPassd/CopyRight2 ==

== system ES105A_StHlthSigNormn/StHlthSigNormn/UpdRawSig/Motor Position 2 /NtcMotPosStHlth/SetNtcSts/CopyRight2 ==

== system ES105A_StHlthSigNormn/StHlthSigNormn/UpdRawSig/Motor Position Error /AbsltMotPosABDifStHlth Calc/If Action Subsystem/CopyRight2 ==

== system ES105A_StHlthSigNormn/StHlthSigNormn/UpdRawSig/Motor Position Error /AbsltMotPosABDifStHlth Calc/If Action Subsystem/If Action Subsystem ==
  Action Port : ActionPort  ActionType=then
  Constant : Constant  Value=HLTH0PERC_CNT_U08  OutDataTypeStr=uint8
  CopyRight2 : Subsystem  Description=|  mask(Copyright Information){none=on}
      | Copyright info block.                                               
      |                                                                     
      | Place copyright information at the top of every subsystem in design.
      mask prompts: none "No parameters"
      mask help: Place copyright information at the top of every subsystem in design.
      mask Display:
      | NxtrConf = 'Nexteer Confidential';
      | 
      | sys = bdroot; %handle for the current model ("system")
      | first = get_param(sys,'Created');
      | first = first(end-3:end);  %year is last four digits
      | 
      | last = get_param(sys,'LastModifiedDate');
      | if isempty(last)
      |     last = datestr(now,'yyyy');
      | else
      |     last = last(end-3:end);
      | end
      | 
      | if strcmp(first,last)
      |     fprintf('%s -- Copyright %s Nexteer',NxtrConf,first)
      | else
      |     fprintf('%s -- %s%s- %s Nexteer',NxtrConf,char(169),first,last)
      | end
  AbsltMotPosABDiffStHlth : Outport
  wires:
  Constant/1 -> AbsltMotPosABDiffStHlth/1
